simulink model "model"  (R2018b)
settings: Solver=VariableStepAuto  StartTime=0.0  StopTime=1  RelTol=1e-3
libraries: Chip_Library x3
settings Model: Creator=phantom  LastModifiedBy=phantom

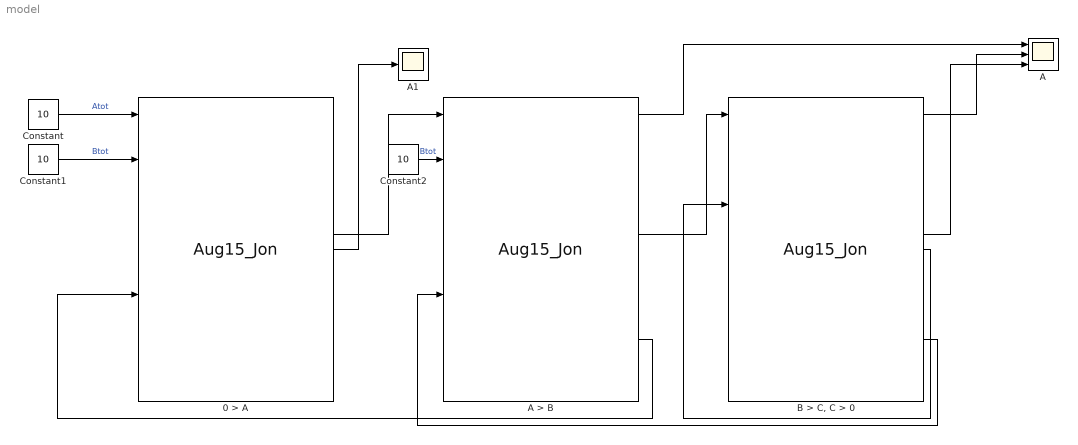
== system model ==
  0 > A : Chip_Library/Aug15_Jon  KDfw=-10  KDrv=10  kr=10  kdeg=1  ratC=0  n=1  c_ic=0.01  A_FB_EN=0  B_FB_EN=0  FF_EN1=0  FF_EN2=1  FF_EN3=1  FF_EN4=0  Ctot_sw=0
  A : Scope  NumInputPorts=3
  A > B : Chip_Library/Aug15_Jon  KDfw=-10  KDrv=20  kr=100  kdeg=1  ratC=0  n=1  c_ic=0.01  A_FB_EN=1  B_FB_EN=0  FF_EN1=0  FF_EN2=1  FF_EN3=1  FF_EN4=0  Ctot_sw=0
  A1 : Scope  NumInputPorts=3
  "B > C, C > 0" : Chip_Library/Aug15_Jon  KDfw=-10  KDrv=20  kr=100  kdeg=1  ratC=1  n=1  c_ic=0.01  A_FB_EN=1  B_FB_EN=0  FF_EN1=0  FF_EN2=1  FF_EN3=1  FF_EN4=0  Ctot_sw=0
  Constant : Constant  Value=10
  Constant1 : Constant  Value=10
  Constant2 : Constant  Value=10
  wires:
  Constant/1 -> 0 > A/1  "Atot"
  Constant1/1 -> 0 > A/2  "Btot"
  0 > A/9 -> A > B/1
  Constant2/1 -> A > B/2  "Btot"
  "B > C, C > 0"/16 -> A > B/5
  A > B/1 -> A/1
  "B > C, C > 0"/1 -> A/2
  "B > C, C > 0"/9 -> A/3
  "B > C, C > 0"/10 -> "B > C, C > 0"/3
  0 > A/10 -> A1/2
  A > B/16 -> 0 > A/5
  A > B/9 -> "B > C, C > 0"/1
